simulink model "my_ODE_block"  (R2021b)
settings: Solver=VariableStepAuto  StartTime=0.0  StopTime=10.0  RelTol=1e-3
settings Model: Creator=Lorenzo  LastModifiedBy=Lorenzo

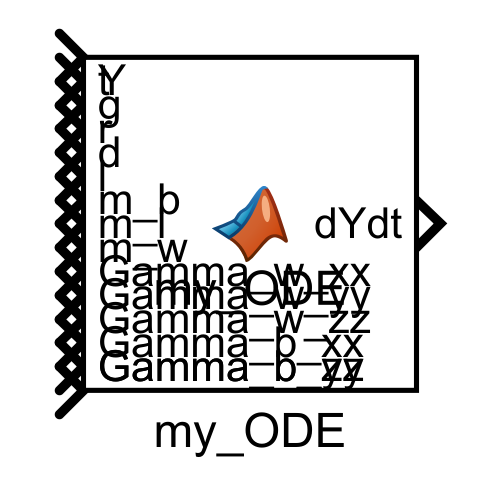
[thumbnail: Simulink's stored preview of the top-level diagram]
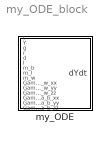
== system my_ODE_block ==
  my_ODE : MATLAB Function  TreatAsAtomicUnit=on

== matlab function my_ODE_block/my_ODE ==
  data: t input; dYdt output; Y input; g input; r input; d input; l input; m_b input; m_l input; m_w input; Gamma_w_xx input; Gamma_w_yy input; Gamma_w_zz input; Gamma_b_xx input; Gamma_b_yy input; Gamma_b_zz input
function dYdt = my_ODE(t,Y,g,r,d,l,m_b,m_l,m_w,Gamma_w_xx,Gamma_w_yy,Gamma_w_zz,Gamma_b_xx,Gamma_b_yy,Gamma_b_zz)
%#codegen

%    This function was generated by the Symbolic Math Toolbox version 9.0.
%    15-Jul-2022 11:26:44

t2 = Gamma_w_yy.^2;
t3 = Y(1);
t4 = Y(2);
t5 = Y(4);
t6 = Y(6);
t7 = d.^2;
t8 = d.^3;
t10 = l.^2;
t11 = m_w.^2;
t12 = m_w.^3;
t13 = r.^2;
t9 = t7.^2;
t14 = t13.^2;
t15 = abs(t4);
t16 = dirac(t4);
t17 = dirac(t5);
t18 = sign(t4);
t19 = sign(t5);
t20 = sin(t3);
t21 = t5.^2;
t22 = t6.^2;
t23 = l.*t4;
t26 = (d.*t5)./2.0;
t24 = t18.^2;
t25 = t19.^3;
t27 = -t26;
t28 = t6+t23;
t33 = t6+t26;
t29 = dirac(t28);
t30 = sign(t28);
t31 = abs(t28);
t34 = sign(t33);
t35 = t6+t27;
t36 = dirac(t33);
t32 = t30.^3;
t37 = sign(t35);
t38 = dirac(t35);
t39 = t6.*t29.*2.0;
t40 = t34.^3;
t42 = t23.*t29.*2.0;
t41 = t37.^3;
t43 = t32+t39+t42;
t44 = Gamma_b_zz.*Gamma_w_yy.*m_w.*t10.*t13.*t25.*t32.*t37.*t40.*4.0;
t46 = Gamma_w_yy.*Gamma_w_zz.*m_w.*t10.*t13.*t25.*t32.*t37.*t40.*8.0;
t49 = Gamma_b_zz.*t10.*t11.*t14.*t25.*t32.*t37.*t40.*4.0;
t51 = Gamma_b_yy.*Gamma_b_zz.*Gamma_w_yy.*t13.*t24.*t25.*t30.*t37.*t40.*4.0;
t53 = Gamma_b_yy.*Gamma_b_zz.*m_w.*t14.*t24.*t25.*t32.*t34.*t37.*4.0;
t54 = Gamma_b_yy.*Gamma_b_zz.*m_w.*t14.*t24.*t25.*t30.*t37.*t40.*4.0;
t56 = Gamma_b_zz.*Gamma_w_yy.*d.*m_w.*t5.*t10.*t13.*t25.*t32.*t36.*t37.*4.0;
t57 = Gamma_b_zz.*Gamma_w_yy.*d.*m_w.*t5.*t10.*t13.*t25.*t32.*t34.*t38.*4.0;
t58 = Gamma_w_zz.*t10.*t11.*t14.*t25.*t32.*t37.*t40.*8.0;
t60 = Gamma_b_yy.*Gamma_w_yy.*Gamma_w_zz.*t13.*t24.*t25.*t30.*t37.*t40.*8.0;
t63 = m_w.*t2.*t9.*t10.*t19.*t21.*t32.*t36.*t38.*4.0;
t64 = Gamma_b_zz.*Gamma_w_yy.*m_w.*t5.*t10.*t13.*t17.*t32.*t37.*t40.*8.0;
t66 = Gamma_b_zz.*Gamma_w_yy.*m_w.*t6.*t10.*t13.*t25.*t32.*t36.*t37.*8.0;
t67 = Gamma_b_zz.*Gamma_w_yy.*m_w.*t6.*t10.*t13.*t25.*t32.*t34.*t38.*8.0;
t68 = Gamma_w_yy.*Gamma_w_zz.*m_w.*t5.*t10.*t13.*t17.*t32.*t37.*t40.*1.6e+1;
t70 = Gamma_w_yy.*Gamma_w_zz.*m_w.*t6.*t10.*t13.*t25.*t32.*t36.*t37.*1.6e+1;
t71 = Gamma_w_yy.*Gamma_w_zz.*m_w.*t6.*t10.*t13.*t25.*t32.*t34.*t38.*1.6e+1;
t73 = m_w.*t2.*t5.*t8.*t10.*t19.*t32.*t38.*t40.*4.0;
t74 = Gamma_b_yy.*Gamma_w_zz.*m_w.*t14.*t24.*t25.*t32.*t34.*t37.*8.0;
t75 = Gamma_b_yy.*Gamma_w_zz.*m_w.*t14.*t24.*t25.*t30.*t37.*t40.*8.0;
t77 = Gamma_b_yy.*Gamma_b_zz.*m_w.*t5.*t14.*t17.*t24.*t32.*t34.*t37.*8.0;
t78 = Gamma_b_yy.*Gamma_b_zz.*m_w.*t5.*t14.*t17.*t24.*t30.*t37.*t40.*8.0;
t80 = Gamma_b_yy.*Gamma_b_zz.*m_w.*t6.*t14.*t24.*t25.*t29.*t34.*t37.*8.0;
t81 = Gamma_b_yy.*Gamma_b_zz.*m_w.*t6.*t14.*t24.*t25.*t30.*t36.*t37.*8.0;
t82 = Gamma_b_yy.*Gamma_b_zz.*m_w.*t6.*t14.*t24.*t25.*t30.*t34.*t38.*8.0;
t83 = Gamma_b_yy.*Gamma_w_zz.*m_w.*t5.*t14.*t17.*t24.*t32.*t34.*t37.*1.6e+1;
t84 = Gamma_b_yy.*Gamma_w_zz.*m_w.*t5.*t14.*t17.*t24.*t30.*t37.*t40.*1.6e+1;
t86 = Gamma_b_yy.*Gamma_w_zz.*m_w.*t6.*t14.*t24.*t25.*t29.*t34.*t37.*1.6e+1;
t87 = Gamma_b_yy.*Gamma_w_zz.*m_w.*t6.*t14.*t24.*t25.*t30.*t36.*t37.*1.6e+1;
t88 = Gamma_b_yy.*Gamma_w_zz.*m_w.*t6.*t14.*t24.*t25.*t30.*t34.*t38.*1.6e+1;
t90 = Gamma_w_yy.*Gamma_w_zz.*d.*m_w.*t5.*t10.*t13.*t25.*t32.*t36.*t37.*8.0;
t91 = Gamma_w_yy.*Gamma_w_zz.*d.*m_w.*t5.*t10.*t13.*t25.*t32.*t34.*t38.*8.0;
t92 = Gamma_b_zz.*d.*t5.*t10.*t11.*t14.*t25.*t32.*t36.*t37.*4.0;
t93 = Gamma_b_zz.*d.*t5.*t10.*t11.*t14.*t25.*t32.*t34.*t38.*4.0;
t94 = Gamma_b_yy.*Gamma_b_zz.*Gamma_w_yy.*d.*t5.*t13.*t24.*t25.*t30.*t36.*t37.*4.0;
t95 = Gamma_b_yy.*Gamma_b_zz.*Gamma_w_yy.*d.*t5.*t13.*t24.*t25.*t30.*t34.*t38.*4.0;
t96 = Gamma_b_yy.*Gamma_b_zz.*d.*m_w.*t5.*t14.*t24.*t25.*t30.*t36.*t37.*4.0;
t97 = Gamma_b_yy.*Gamma_b_zz.*d.*m_w.*t5.*t14.*t24.*t25.*t30.*t34.*t38.*4.0;
t98 = Gamma_b_yy.*Gamma_w_yy.*m_w.*t7.*t13.*t19.*t24.*t32.*t37.*t40;
t101 = m_w.*t2.*t7.*t10.*t19.*t22.*t32.*t36.*t38.*1.6e+1;
t104 = m_w.*t2.*t6.*t7.*t10.*t19.*t32.*t38.*t40.*8.0;
t105 = Gamma_b_zz.*t5.*t10.*t11.*t14.*t17.*t32.*t37.*t40.*8.0;
t107 = Gamma_b_zz.*t6.*t10.*t11.*t14.*t25.*t32.*t36.*t37.*8.0;
t108 = Gamma_b_zz.*t6.*t10.*t11.*t14.*t25.*t32.*t34.*t38.*8.0;
t109 = Gamma_w_zz.*t5.*t10.*t11.*t14.*t17.*t32.*t37.*t40.*1.6e+1;
t111 = Gamma_w_zz.*t6.*t10.*t11.*t14.*t25.*t32.*t36.*t37.*1.6e+1;
t112 = Gamma_w_zz.*t6.*t10.*t11.*t14.*t25.*t32.*t34.*t38.*1.6e+1;
t113 = Gamma_b_yy.*t2.*t9.*t19.*t21.*t24.*t30.*t36.*t38.*4.0;
t114 = Gamma_b_yy.*Gamma_b_zz.*Gamma_w_yy.*t5.*t13.*t17.*t24.*t30.*t37.*t40.*8.0;
t116 = Gamma_b_yy.*Gamma_b_zz.*Gamma_w_yy.*t6.*t13.*t24.*t25.*t30.*t36.*t37.*8.0;
t117 = Gamma_b_yy.*Gamma_b_zz.*Gamma_w_yy.*t6.*t13.*t24.*t25.*t30.*t34.*t38.*8.0;
t118 = Gamma_b_yy.*Gamma_w_yy.*Gamma_w_zz.*t5.*t13.*t17.*t24.*t30.*t37.*t40.*1.6e+1;
t120 = Gamma_b_yy.*Gamma_w_yy.*Gamma_w_zz.*t6.*t13.*t24.*t25.*t30.*t36.*t37.*1.6e+1;
t121 = Gamma_b_yy.*Gamma_w_yy.*Gamma_w_zz.*t6.*t13.*t24.*t25.*t30.*t34.*t38.*1.6e+1;
t123 = Gamma_b_yy.*t2.*t5.*t8.*t19.*t24.*t30.*t38.*t40.*4.0;
t124 = Gamma_b_zz.*Gamma_w_yy.*m_w.*t5.*t6.*t10.*t13.*t17.*t32.*t36.*t37.*1.6e+1;
t125 = Gamma_b_zz.*Gamma_w_yy.*m_w.*t5.*t6.*t10.*t13.*t17.*t32.*t34.*t38.*1.6e+1;
t126 = Gamma_w_yy.*Gamma_w_zz.*m_w.*t5.*t6.*t10.*t13.*t17.*t32.*t36.*t37.*3.2e+1;
t127 = Gamma_w_yy.*Gamma_w_zz.*m_w.*t5.*t6.*t10.*t13.*t17.*t32.*t34.*t38.*3.2e+1;
t129 = Gamma_b_zz.*Gamma_w_yy.*d.*m_w.*t10.*t13.*t17.*t21.*t32.*t36.*t37.*8.0;
t130 = Gamma_b_zz.*Gamma_w_yy.*d.*m_w.*t10.*t13.*t17.*t21.*t32.*t34.*t38.*8.0;
t131 = Gamma_w_yy.*Gamma_w_zz.*d.*m_w.*t10.*t13.*t17.*t21.*t32.*t36.*t37.*1.6e+1;
t132 = Gamma_w_yy.*Gamma_w_zz.*d.*m_w.*t10.*t13.*t17.*t21.*t32.*t34.*t38.*1.6e+1;
t133 = Gamma_b_zz.*t5.*t6.*t10.*t11.*t14.*t17.*t32.*t36.*t37.*1.6e+1;
t134 = Gamma_b_zz.*t5.*t6.*t10.*t11.*t14.*t17.*t32.*t34.*t38.*1.6e+1;
t135 = Gamma_w_zz.*t5.*t6.*t10.*t11.*t14.*t17.*t32.*t36.*t37.*3.2e+1;
t136 = Gamma_w_zz.*t5.*t6.*t10.*t11.*t14.*t17.*t32.*t34.*t38.*3.2e+1;
t138 = Gamma_b_zz.*d.*t10.*t11.*t14.*t17.*t21.*t32.*t36.*t37.*8.0;
t139 = Gamma_b_zz.*d.*t10.*t11.*t14.*t17.*t21.*t32.*t34.*t38.*8.0;
t140 = Gamma_w_zz.*d.*t10.*t11.*t14.*t17.*t21.*t32.*t36.*t37.*1.6e+1;
t141 = Gamma_w_zz.*d.*t10.*t11.*t14.*t17.*t21.*t32.*t34.*t38.*1.6e+1;
t143 = Gamma_w_zz.*d.*t5.*t10.*t11.*t14.*t25.*t32.*t36.*t37.*8.0;
t144 = Gamma_w_zz.*d.*t5.*t10.*t11.*t14.*t25.*t32.*t34.*t38.*8.0;
t145 = Gamma_b_yy.*Gamma_b_zz.*Gamma_w_yy.*t5.*t6.*t13.*t17.*t24.*t30.*t36.*t37.*1.6e+1;
t146 = Gamma_b_yy.*Gamma_b_zz.*Gamma_w_yy.*t5.*t6.*t13.*t17.*t24.*t30.*t34.*t38.*1.6e+1;
t147 = Gamma_b_yy.*Gamma_w_yy.*Gamma_w_zz.*t5.*t6.*t13.*t17.*t24.*t30.*t36.*t37.*3.2e+1;
t148 = Gamma_b_yy.*Gamma_w_yy.*Gamma_w_zz.*t5.*t6.*t13.*t17.*t24.*t30.*t34.*t38.*3.2e+1;
t149 = t9.*t10.*t12.*t14.*t19.*t21.*t32.*t36.*t38.*4.0;
t150 = Gamma_b_yy.*Gamma_b_zz.*Gamma_w_yy.*d.*t13.*t17.*t21.*t24.*t30.*t36.*t37.*8.0;
t151 = Gamma_b_yy.*Gamma_b_zz.*Gamma_w_yy.*d.*t13.*t17.*t21.*t24.*t30.*t34.*t38.*8.0;
t152 = Gamma_b_yy.*Gamma_w_yy.*Gamma_w_zz.*d.*t13.*t17.*t21.*t24.*t30.*t36.*t37.*1.6e+1;
t153 = Gamma_b_yy.*Gamma_w_yy.*Gamma_w_zz.*d.*t13.*t17.*t21.*t24.*t30.*t34.*t38.*1.6e+1;
t155 = t5.*t8.*t10.*t12.*t14.*t19.*t32.*t38.*t40.*4.0;
t156 = Gamma_b_yy.*Gamma_b_zz.*Gamma_w_yy.*t13.*t15.*t16.*t25.*t30.*t37.*t40.*8.0;
t158 = Gamma_b_yy.*Gamma_w_yy.*Gamma_w_zz.*t13.*t15.*t16.*t25.*t30.*t37.*t40.*1.6e+1;
t161 = Gamma_b_yy.*Gamma_w_yy.*Gamma_w_zz.*d.*t5.*t13.*t24.*t25.*t30.*t36.*t37.*8.0;
t162 = Gamma_b_yy.*Gamma_w_yy.*Gamma_w_zz.*d.*t5.*t13.*t24.*t25.*t30.*t34.*t38.*8.0;
t163 = Gamma_b_yy.*Gamma_b_zz.*m_w.*t5.*t6.*t14.*t17.*t24.*t29.*t34.*t37.*1.6e+1;
t164 = Gamma_b_yy.*Gamma_b_zz.*m_w.*t5.*t6.*t14.*t17.*t24.*t30.*t36.*t37.*1.6e+1;
t165 = Gamma_b_yy.*Gamma_b_zz.*m_w.*t5.*t6.*t14.*t17.*t24.*t30.*t34.*t38.*1.6e+1;
t166 = Gamma_b_yy.*Gamma_w_zz.*m_w.*t5.*t6.*t14.*t17.*t24.*t29.*t34.*t37.*3.2e+1;
t167 = Gamma_b_yy.*Gamma_w_zz.*m_w.*t5.*t6.*t14.*t17.*t24.*t30.*t36.*t37.*3.2e+1;
t168 = Gamma_b_yy.*Gamma_w_zz.*m_w.*t5.*t6.*t14.*t17.*t24.*t30.*t34.*t38.*3.2e+1;
t169 = Gamma_b_yy.*Gamma_b_zz.*d.*m_w.*t14.*t17.*t21.*t24.*t30.*t36.*t37.*8.0;
t170 = Gamma_b_yy.*Gamma_b_zz.*d.*m_w.*t14.*t17.*t21.*t24.*t30.*t34.*t38.*8.0;
t171 = Gamma_b_yy.*Gamma_w_zz.*d.*m_w.*t14.*t17.*t21.*t24.*t30.*t36.*t37.*1.6e+1;
t172 = Gamma_b_yy.*Gamma_w_zz.*d.*m_w.*t14.*t17.*t21.*t24.*t30.*t34.*t38.*1.6e+1;
t173 = Gamma_b_yy.*Gamma_b_zz.*m_w.*t14.*t15.*t16.*t25.*t32.*t34.*t37.*8.0;
t174 = Gamma_b_yy.*Gamma_b_zz.*m_w.*t14.*t15.*t16.*t25.*t30.*t37.*t40.*8.0;
t176 = Gamma_b_yy.*Gamma_w_zz.*m_w.*t14.*t15.*t16.*t25.*t32.*t34.*t37.*1.6e+1;
t177 = Gamma_b_yy.*Gamma_w_zz.*m_w.*t14.*t15.*t16.*t25.*t30.*t37.*t40.*1.6e+1;
t180 = Gamma_b_yy.*Gamma_w_zz.*d.*m_w.*t5.*t14.*t24.*t25.*t30.*t36.*t37.*8.0;
t181 = Gamma_b_yy.*Gamma_w_zz.*d.*m_w.*t5.*t14.*t24.*t25.*t30.*t34.*t38.*8.0;
t182 = Gamma_b_yy.*Gamma_b_zz.*m_w.*t14.*t23.*t24.*t25.*t29.*t34.*t37.*8.0;
t183 = Gamma_b_yy.*Gamma_w_zz.*m_w.*t14.*t23.*t24.*t25.*t29.*t34.*t37.*1.6e+1;
t184 = Gamma_b_yy.*t7.*t11.*t14.*t19.*t24.*t32.*t37.*t40;
t186 = Gamma_b_yy.*Gamma_w_yy.*m_w.*t5.*t8.*t13.*t19.*t24.*t32.*t36.*t37;
t187 = Gamma_b_yy.*Gamma_w_yy.*m_w.*t5.*t8.*t13.*t19.*t24.*t32.*t34.*t38;
t189 = Gamma_b_yy.*t2.*t7.*t19.*t22.*t24.*t30.*t36.*t38.*1.6e+1;
t192 = Gamma_b_yy.*t2.*t6.*t7.*t19.*t24.*t30.*t38.*t40.*8.0;
t199 = t7.*t10.*t12.*t14.*t19.*t22.*t32.*t36.*t38.*1.6e+1;
t205 = t6.*t7.*t10.*t12.*t14.*t19.*t32.*t38.*t40.*8.0;
t212 = Gamma_b_yy.*Gamma_b_zz.*Gamma_w_yy.*t5.*t13.*t15.*t16.*t17.*t30.*t37.*t40.*1.6e+1;
t214 = Gamma_b_yy.*Gamma_b_zz.*Gamma_w_yy.*t6.*t13.*t15.*t16.*t25.*t30.*t36.*t37.*1.6e+1;
t215 = Gamma_b_yy.*Gamma_b_zz.*Gamma_w_yy.*t6.*t13.*t15.*t16.*t25.*t30.*t34.*t38.*1.6e+1;
t216 = Gamma_b_yy.*Gamma_w_yy.*Gamma_w_zz.*t5.*t13.*t15.*t16.*t17.*t30.*t37.*t40.*3.2e+1;
t218 = Gamma_b_yy.*Gamma_w_yy.*Gamma_w_zz.*t6.*t13.*t15.*t16.*t25.*t30.*t36.*t37.*3.2e+1;
t219 = Gamma_b_yy.*Gamma_w_yy.*Gamma_w_zz.*t6.*t13.*t15.*t16.*t25.*t30.*t34.*t38.*3.2e+1;
t221 = Gamma_b_yy.*Gamma_b_zz.*m_w.*t5.*t14.*t15.*t16.*t17.*t32.*t34.*t37.*1.6e+1;
t222 = Gamma_b_yy.*Gamma_b_zz.*m_w.*t5.*t14.*t15.*t16.*t17.*t30.*t37.*t40.*1.6e+1;
t224 = Gamma_b_yy.*Gamma_b_zz.*m_w.*t6.*t14.*t15.*t16.*t25.*t29.*t34.*t37.*1.6e+1;
t225 = Gamma_b_yy.*Gamma_b_zz.*m_w.*t6.*t14.*t15.*t16.*t25.*t30.*t36.*t37.*1.6e+1;
t226 = Gamma_b_yy.*Gamma_b_zz.*m_w.*t6.*t14.*t15.*t16.*t25.*t30.*t34.*t38.*1.6e+1;
t227 = Gamma_b_yy.*Gamma_w_zz.*m_w.*t5.*t14.*t15.*t16.*t17.*t32.*t34.*t37.*3.2e+1;
t228 = Gamma_b_yy.*Gamma_w_zz.*m_w.*t5.*t14.*t15.*t16.*t17.*t30.*t37.*t40.*3.2e+1;
t230 = Gamma_b_yy.*Gamma_w_zz.*m_w.*t6.*t14.*t15.*t16.*t25.*t29.*t34.*t37.*3.2e+1;
t231 = Gamma_b_yy.*Gamma_w_zz.*m_w.*t6.*t14.*t15.*t16.*t25.*t30.*t36.*t37.*3.2e+1;
t232 = Gamma_b_yy.*Gamma_w_zz.*m_w.*t6.*t14.*t15.*t16.*t25.*t30.*t34.*t38.*3.2e+1;
t233 = Gamma_b_yy.*Gamma_w_yy.*m_w.*t7.*t13.*t19.*t22.*t24.*t29.*t36.*t37.*4.0;
t234 = Gamma_b_yy.*Gamma_w_yy.*m_w.*t7.*t13.*t19.*t22.*t24.*t29.*t34.*t38.*4.0;
t235 = Gamma_b_yy.*Gamma_b_zz.*m_w.*t5.*t14.*t17.*t23.*t24.*t29.*t34.*t37.*1.6e+1;
t236 = Gamma_b_yy.*Gamma_w_zz.*m_w.*t5.*t14.*t17.*t23.*t24.*t29.*t34.*t37.*3.2e+1;
t237 = Gamma_b_yy.*Gamma_w_yy.*m_w.*t7.*t13.*t19.*t24.*t37.*t39.*t40;
t239 = Gamma_b_yy.*Gamma_w_yy.*m_w.*t6.*t7.*t13.*t19.*t24.*t32.*t36.*t37.*2.0;
t240 = Gamma_b_yy.*Gamma_w_yy.*m_w.*t6.*t7.*t13.*t19.*t24.*t32.*t34.*t38.*2.0;
t241 = Gamma_b_yy.*t5.*t8.*t11.*t14.*t19.*t24.*t32.*t36.*t37;
t242 = Gamma_b_yy.*t5.*t8.*t11.*t14.*t19.*t24.*t32.*t34.*t38;
t243 = Gamma_b_yy.*Gamma_b_zz.*d.*m_w.*t14.*t15.*t16.*t17.*t21.*t30.*t36.*t37.*1.6e+1;
t244 = Gamma_b_yy.*Gamma_b_zz.*d.*m_w.*t14.*t15.*t16.*t17.*t21.*t30.*t34.*t38.*1.6e+1;
t245 = Gamma_b_yy.*Gamma_w_zz.*d.*m_w.*t14.*t15.*t16.*t17.*t21.*t30.*t36.*t37.*3.2e+1;
t246 = Gamma_b_yy.*Gamma_w_zz.*d.*m_w.*t14.*t15.*t16.*t17.*t21.*t30.*t34.*t38.*3.2e+1;
t247 = Gamma_b_yy.*Gamma_w_yy.*m_w.*t5.*t8.*t13.*t19.*t24.*t36.*t37.*t39;
t248 = Gamma_b_yy.*Gamma_w_yy.*m_w.*t5.*t8.*t13.*t19.*t24.*t34.*t38.*t39;
t249 = Gamma_b_yy.*Gamma_b_zz.*d.*m_w.*t5.*t14.*t15.*t16.*t25.*t30.*t36.*t37.*8.0;
t250 = Gamma_b_yy.*Gamma_b_zz.*d.*m_w.*t5.*t14.*t15.*t16.*t25.*t30.*t34.*t38.*8.0;
t251 = Gamma_b_yy.*Gamma_w_zz.*d.*m_w.*t5.*t14.*t15.*t16.*t25.*t30.*t36.*t37.*1.6e+1;
t252 = Gamma_b_yy.*Gamma_w_zz.*d.*m_w.*t5.*t14.*t15.*t16.*t25.*t30.*t34.*t38.*1.6e+1;
t253 = Gamma_b_yy.*Gamma_b_zz.*m_w.*t14.*t15.*t16.*t23.*t25.*t29.*t34.*t37.*1.6e+1;
t254 = Gamma_b_yy.*Gamma_w_zz.*m_w.*t14.*t15.*t16.*t23.*t25.*t29.*t34.*t37.*3.2e+1;
t255 = Gamma_b_yy.*Gamma_w_yy.*m_w.*t7.*t13.*t15.*t16.*t19.*t32.*t37.*t40.*2.0;
t257 = Gamma_b_yy.*Gamma_w_yy.*m_w.*t7.*t13.*t19.*t24.*t37.*t40.*t42;
t259 = Gamma_w_yy.*t9.*t10.*t11.*t13.*t19.*t21.*t32.*t36.*t38.*8.0;
t260 = Gamma_w_yy.*t7.*t10.*t11.*t13.*t19.*t22.*t32.*t36.*t38.*3.2e+1;
t262 = Gamma_w_yy.*t5.*t8.*t10.*t11.*t13.*t19.*t32.*t38.*t40.*8.0;
t264 = Gamma_w_yy.*t6.*t7.*t10.*t11.*t13.*t19.*t32.*t38.*t40.*1.6e+1;
t265 = Gamma_b_yy.*t2.*t9.*t15.*t16.*t19.*t21.*t30.*t36.*t38.*8.0;
t266 = Gamma_b_yy.*t2.*t7.*t15.*t16.*t19.*t22.*t30.*t36.*t38.*3.2e+1;
t268 = Gamma_b_yy.*t2.*t5.*t8.*t15.*t16.*t19.*t30.*t38.*t40.*8.0;
t270 = Gamma_b_yy.*t2.*t6.*t7.*t15.*t16.*t19.*t30.*t38.*t40.*1.6e+1;
t271 = Gamma_b_yy.*Gamma_w_yy.*m_w.*t9.*t13.*t19.*t21.*t24.*t30.*t36.*t38.*8.0;
t272 = Gamma_b_yy.*Gamma_w_yy.*m_w.*t7.*t13.*t19.*t22.*t24.*t30.*t36.*t38.*3.2e+1;
t275 = Gamma_b_yy.*Gamma_w_yy.*m_w.*t5.*t8.*t13.*t19.*t24.*t30.*t38.*t40.*8.0;
t277 = Gamma_b_yy.*Gamma_w_yy.*m_w.*t6.*t7.*t13.*t19.*t24.*t30.*t38.*t40.*1.6e+1;
t278 = Gamma_b_yy.*t7.*t11.*t14.*t19.*t22.*t24.*t29.*t36.*t37.*4.0;
t279 = Gamma_b_yy.*t7.*t11.*t14.*t19.*t22.*t24.*t29.*t34.*t38.*4.0;
t280 = Gamma_b_yy.*t9.*t11.*t14.*t19.*t21.*t24.*t30.*t36.*t38.*4.0;
t281 = Gamma_b_yy.*Gamma_b_zz.*Gamma_w_yy.*t5.*t6.*t13.*t15.*t16.*t17.*t30.*t36.*t37.*3.2e+1;
t282 = Gamma_b_yy.*Gamma_b_zz.*Gamma_w_yy.*t5.*t6.*t13.*t15.*t16.*t17.*t30.*t34.*t38.*3.2e+1;
t283 = Gamma_b_yy.*Gamma_b_zz.*Gamma_w_yy.*d.*t13.*t15.*t16.*t17.*t21.*t30.*t36.*t37.*1.6e+1;
t284 = Gamma_b_yy.*Gamma_b_zz.*Gamma_w_yy.*d.*t13.*t15.*t16.*t17.*t21.*t30.*t34.*t38.*1.6e+1;
t285 = Gamma_b_yy.*Gamma_w_yy.*Gamma_w_zz.*d.*t13.*t15.*t16.*t17.*t21.*t30.*t36.*t37.*3.2e+1;
t286 = Gamma_b_yy.*Gamma_w_yy.*Gamma_w_zz.*d.*t13.*t15.*t16.*t17.*t21.*t30.*t34.*t38.*3.2e+1;
t287 = Gamma_b_yy.*t7.*t11.*t14.*t19.*t24.*t37.*t39.*t40;
t289 = Gamma_b_yy.*t6.*t7.*t11.*t14.*t19.*t24.*t32.*t36.*t37.*2.0;
t290 = Gamma_b_yy.*t6.*t7.*t11.*t14.*t19.*t24.*t32.*t34.*t38.*2.0;
t292 = Gamma_b_yy.*t5.*t8.*t11.*t14.*t19.*t24.*t30.*t38.*t40.*4.0;
t293 = Gamma_b_yy.*Gamma_b_zz.*Gamma_w_yy.*d.*t5.*t13.*t15.*t16.*t25.*t30.*t36.*t37.*8.0;
t294 = Gamma_b_yy.*Gamma_b_zz.*Gamma_w_yy.*d.*t5.*t13.*t15.*t16.*t25.*t30.*t34.*t38.*8.0;
t295 = Gamma_b_yy.*Gamma_w_yy.*Gamma_w_zz.*d.*t5.*t13.*t15.*t16.*t25.*t30.*t36.*t37.*1.6e+1;
t296 = Gamma_b_yy.*Gamma_w_yy.*Gamma_w_zz.*d.*t5.*t13.*t15.*t16.*t25.*t30.*t34.*t38.*1.6e+1;
t297 = Gamma_b_yy.*Gamma_b_zz.*m_w.*t5.*t6.*t14.*t15.*t16.*t17.*t29.*t34.*t37.*3.2e+1;
t298 = Gamma_b_yy.*Gamma_b_zz.*m_w.*t5.*t6.*t14.*t15.*t16.*t17.*t30.*t36.*t37.*3.2e+1;
t299 = Gamma_b_yy.*Gamma_b_zz.*m_w.*t5.*t6.*t14.*t15.*t16.*t17.*t30.*t34.*t38.*3.2e+1;
t302 = Gamma_b_yy.*Gamma_w_yy.*m_w.*t5.*t6.*t8.*t13.*t19.*t24.*t29.*t34.*t38.*-2.0;
t306 = Gamma_b_yy.*t5.*t8.*t11.*t14.*t19.*t24.*t36.*t37.*t39;
t307 = Gamma_b_yy.*t5.*t8.*t11.*t14.*t19.*t24.*t34.*t38.*t39;
t308 = Gamma_b_yy.*t7.*t11.*t14.*t15.*t16.*t19.*t32.*t37.*t40.*2.0;
t310 = Gamma_b_yy.*t7.*t11.*t14.*t19.*t24.*t37.*t40.*t42;
t312 = Gamma_b_yy.*Gamma_b_zz.*m_w.*t5.*t14.*t15.*t16.*t17.*t23.*t29.*t34.*t37.*3.2e+1;
t314 = Gamma_b_yy.*Gamma_w_yy.*m_w.*t5.*t8.*t13.*t15.*t16.*t19.*t32.*t36.*t37.*2.0;
t315 = Gamma_b_yy.*Gamma_w_yy.*m_w.*t5.*t8.*t13.*t15.*t16.*t19.*t32.*t34.*t38.*2.0;
t316 = Gamma_b_yy.*Gamma_w_yy.*m_w.*t6.*t7.*t13.*t15.*t16.*t19.*t29.*t37.*t40.*4.0;
t318 = Gamma_b_yy.*Gamma_w_yy.*m_w.*t6.*t7.*t13.*t15.*t16.*t19.*t32.*t36.*t37.*4.0;
t319 = Gamma_b_yy.*Gamma_w_yy.*m_w.*t6.*t7.*t13.*t15.*t16.*t19.*t32.*t34.*t38.*4.0;
t320 = Gamma_b_yy.*Gamma_w_yy.*m_w.*t5.*t8.*t13.*t19.*t24.*t36.*t37.*t42;
t321 = Gamma_b_yy.*Gamma_w_yy.*m_w.*t5.*t8.*t13.*t19.*t24.*t34.*t38.*t42;
t322 = Gamma_b_yy.*Gamma_w_yy.*m_w.*t6.*t7.*t13.*t19.*t23.*t24.*t29.*t36.*t37.*4.0;
t323 = Gamma_b_yy.*Gamma_w_yy.*m_w.*t6.*t7.*t13.*t19.*t23.*t24.*t29.*t34.*t38.*4.0;
t330 = Gamma_b_yy.*t7.*t11.*t14.*t19.*t22.*t24.*t30.*t36.*t38.*1.6e+1;
t331 = Gamma_b_yy.*Gamma_w_yy.*Gamma_w_zz.*t5.*t6.*t13.*t15.*t16.*t17.*t30.*t36.*t37.*6.4e+1;
t332 = Gamma_b_yy.*Gamma_w_yy.*Gamma_w_zz.*t5.*t6.*t13.*t15.*t16.*t17.*t30.*t34.*t38.*6.4e+1;
t338 = Gamma_b_yy.*t6.*t7.*t11.*t14.*t19.*t24.*t30.*t38.*t40.*8.0;
t341 = Gamma_b_yy.*Gamma_w_zz.*m_w.*t5.*t6.*t14.*t15.*t16.*t17.*t29.*t34.*t37.*6.4e+1;
t342 = Gamma_b_yy.*Gamma_w_zz.*m_w.*t5.*t6.*t14.*t15.*t16.*t17.*t30.*t36.*t37.*6.4e+1;
t343 = Gamma_b_yy.*Gamma_w_zz.*m_w.*t5.*t6.*t14.*t15.*t16.*t17.*t30.*t34.*t38.*6.4e+1;
t344 = Gamma_b_yy.*t5.*t6.*t8.*t11.*t14.*t19.*t24.*t29.*t34.*t38.*-2.0;
t346 = Gamma_b_yy.*Gamma_w_yy.*m_w.*t7.*t13.*t15.*t16.*t19.*t22.*t29.*t36.*t37.*8.0;
t347 = Gamma_b_yy.*Gamma_w_yy.*m_w.*t7.*t13.*t15.*t16.*t19.*t22.*t29.*t34.*t38.*8.0;
t348 = Gamma_b_yy.*Gamma_w_yy.*m_w.*t9.*t13.*t15.*t16.*t19.*t21.*t30.*t36.*t38.*1.6e+1;
t349 = Gamma_b_yy.*Gamma_w_zz.*m_w.*t5.*t14.*t15.*t16.*t17.*t23.*t29.*t34.*t37.*6.4e+1;
t352 = Gamma_b_yy.*Gamma_w_yy.*m_w.*t5.*t8.*t13.*t15.*t16.*t19.*t30.*t38.*t40.*1.6e+1;
t354 = Gamma_b_yy.*Gamma_w_yy.*m_w.*t6.*t7.*t13.*t15.*t16.*t19.*t30.*t38.*t40.*3.2e+1;
t355 = Gamma_b_yy.*Gamma_w_yy.*m_w.*t5.*t8.*t13.*t19.*t23.*t24.*t29.*t34.*t38.*-2.0;
t356 = Gamma_b_yy.*t5.*t8.*t11.*t14.*t15.*t16.*t19.*t32.*t36.*t37.*2.0;
t357 = Gamma_b_yy.*t5.*t8.*t11.*t14.*t15.*t16.*t19.*t32.*t34.*t38.*2.0;
t358 = Gamma_b_yy.*t6.*t7.*t11.*t14.*t15.*t16.*t19.*t29.*t37.*t40.*4.0;
t360 = Gamma_b_yy.*t6.*t7.*t11.*t14.*t15.*t16.*t19.*t32.*t36.*t37.*4.0;
t361 = Gamma_b_yy.*t6.*t7.*t11.*t14.*t15.*t16.*t19.*t32.*t34.*t38.*4.0;
t362 = Gamma_b_yy.*t5.*t8.*t11.*t14.*t19.*t24.*t36.*t37.*t42;
t363 = Gamma_b_yy.*t5.*t8.*t11.*t14.*t19.*t24.*t34.*t38.*t42;
t364 = Gamma_b_yy.*t6.*t7.*t11.*t14.*t19.*t23.*t24.*t29.*t36.*t37.*4.0;
t365 = Gamma_b_yy.*t6.*t7.*t11.*t14.*t19.*t23.*t24.*t29.*t34.*t38.*4.0;
t366 = Gamma_b_yy.*Gamma_w_yy.*m_w.*t5.*t6.*t8.*t13.*t15.*t16.*t19.*t29.*t36.*t37.*4.0;
t367 = Gamma_b_yy.*Gamma_w_yy.*m_w.*t5.*t6.*t8.*t13.*t15.*t16.*t19.*t29.*t34.*t38.*4.0;
t368 = Gamma_b_yy.*Gamma_w_yy.*m_w.*t7.*t13.*t15.*t16.*t19.*t23.*t29.*t37.*t40.*4.0;
t370 = Gamma_b_yy.*Gamma_w_yy.*m_w.*t5.*t8.*t13.*t15.*t16.*t19.*t23.*t29.*t36.*t37.*4.0;
t371 = Gamma_b_yy.*Gamma_w_yy.*m_w.*t5.*t8.*t13.*t15.*t16.*t19.*t23.*t29.*t34.*t38.*4.0;
t373 = Gamma_b_yy.*Gamma_w_yy.*m_w.*t7.*t13.*t15.*t16.*t19.*t22.*t30.*t36.*t38.*6.4e+1;
t375 = Gamma_b_yy.*t7.*t11.*t14.*t15.*t16.*t19.*t22.*t29.*t36.*t37.*8.0;
t376 = Gamma_b_yy.*t7.*t11.*t14.*t15.*t16.*t19.*t22.*t29.*t34.*t38.*8.0;
t377 = Gamma_b_yy.*t9.*t11.*t14.*t15.*t16.*t19.*t21.*t30.*t36.*t38.*8.0;
t378 = Gamma_b_yy.*t7.*t11.*t14.*t15.*t16.*t19.*t22.*t30.*t36.*t38.*3.2e+1;
t381 = Gamma_b_yy.*t5.*t8.*t11.*t14.*t15.*t16.*t19.*t30.*t38.*t40.*8.0;
t383 = Gamma_b_yy.*t6.*t7.*t11.*t14.*t15.*t16.*t19.*t30.*t38.*t40.*1.6e+1;
t384 = Gamma_b_yy.*t5.*t8.*t11.*t14.*t19.*t23.*t24.*t29.*t34.*t38.*-2.0;
t386 = Gamma_b_yy.*t5.*t6.*t8.*t11.*t14.*t15.*t16.*t19.*t29.*t36.*t37.*4.0;
t387 = Gamma_b_yy.*t5.*t6.*t8.*t11.*t14.*t15.*t16.*t19.*t29.*t34.*t38.*4.0;
t388 = Gamma_b_yy.*t7.*t11.*t14.*t15.*t16.*t19.*t23.*t29.*t37.*t40.*4.0;
t391 = Gamma_b_yy.*Gamma_w_yy.*m_w.*t6.*t7.*t13.*t15.*t16.*t19.*t23.*t29.*t36.*t37.*8.0;
t392 = Gamma_b_yy.*Gamma_w_yy.*m_w.*t6.*t7.*t13.*t15.*t16.*t19.*t23.*t29.*t34.*t38.*8.0;
t393 = Gamma_b_yy.*t5.*t8.*t11.*t14.*t15.*t16.*t19.*t23.*t29.*t36.*t37.*4.0;
t394 = Gamma_b_yy.*t5.*t8.*t11.*t14.*t15.*t16.*t19.*t23.*t29.*t34.*t38.*4.0;
t399 = Gamma_b_yy.*t6.*t7.*t11.*t14.*t15.*t16.*t19.*t23.*t29.*t36.*t37.*8.0;
t400 = Gamma_b_yy.*t6.*t7.*t11.*t14.*t15.*t16.*t19.*t23.*t29.*t34.*t38.*8.0;
t401 = Gamma_b_zz.*Gamma_w_yy.*m_w.*t10.*t13.*t25.*t29.*t30.*t31.*t37.*t40.*8.0;
t403 = Gamma_w_yy.*Gamma_w_zz.*m_w.*t10.*t13.*t25.*t29.*t30.*t31.*t37.*t40.*1.6e+1;
t406 = Gamma_b_zz.*t10.*t11.*t14.*t25.*t29.*t30.*t31.*t37.*t40.*8.0;
t408 = Gamma_w_zz.*t10.*t11.*t14.*t25.*t29.*t30.*t31.*t37.*t40.*1.6e+1;
t410 = Gamma_b_zz.*Gamma_w_yy.*m_w.*t5.*t10.*t13.*t17.*t29.*t30.*t31.*t37.*t40.*1.6e+1;
t412 = Gamma_b_zz.*Gamma_w_yy.*m_w.*t6.*t10.*t13.*t25.*t29.*t30.*t31.*t36.*t37.*1.6e+1;
t413 = Gamma_b_zz.*Gamma_w_yy.*m_w.*t6.*t10.*t13.*t25.*t29.*t30.*t31.*t34.*t38.*1.6e+1;
t414 = Gamma_w_yy.*Gamma_w_zz.*m_w.*t5.*t10.*t13.*t17.*t29.*t30.*t31.*t37.*t40.*3.2e+1;
t416 = Gamma_w_yy.*Gamma_w_zz.*m_w.*t6.*t10.*t13.*t25.*t29.*t30.*t31.*t36.*t37.*3.2e+1;
t417 = Gamma_w_yy.*Gamma_w_zz.*m_w.*t6.*t10.*t13.*t25.*t29.*t30.*t31.*t34.*t38.*3.2e+1;
t418 = m_w.*t2.*t9.*t10.*t19.*t21.*t29.*t30.*t31.*t36.*t38.*8.0;
t419 = m_w.*t2.*t7.*t10.*t19.*t22.*t29.*t30.*t31.*t36.*t38.*3.2e+1;
t421 = m_w.*t2.*t5.*t8.*t10.*t19.*t29.*t30.*t31.*t38.*t40.*8.0;
t423 = m_w.*t2.*t6.*t7.*t10.*t19.*t29.*t30.*t31.*t38.*t40.*1.6e+1;
t424 = Gamma_b_zz.*t5.*t10.*t11.*t14.*t17.*t29.*t30.*t31.*t37.*t40.*1.6e+1;
t426 = Gamma_b_zz.*t6.*t10.*t11.*t14.*t25.*t29.*t30.*t31.*t36.*t37.*1.6e+1;
t427 = Gamma_b_zz.*t6.*t10.*t11.*t14.*t25.*t29.*t30.*t31.*t34.*t38.*1.6e+1;
t428 = Gamma_w_zz.*t5.*t10.*t11.*t14.*t17.*t29.*t30.*t31.*t37.*t40.*3.2e+1;
t430 = Gamma_w_zz.*t6.*t10.*t11.*t14.*t25.*t29.*t30.*t31.*t36.*t37.*3.2e+1;
t431 = Gamma_w_zz.*t6.*t10.*t11.*t14.*t25.*t29.*t30.*t31.*t34.*t38.*3.2e+1;
t432 = Gamma_b_zz.*Gamma_w_yy.*m_w.*t5.*t6.*t10.*t13.*t17.*t29.*t30.*t31.*t36.*t37.*3.2e+1;
t433 = Gamma_b_zz.*Gamma_w_yy.*m_w.*t5.*t6.*t10.*t13.*t17.*t29.*t30.*t31.*t34.*t38.*3.2e+1;
t434 = Gamma_b_zz.*Gamma_w_yy.*d.*m_w.*t10.*t13.*t17.*t21.*t29.*t30.*t31.*t36.*t37.*1.6e+1;
t435 = Gamma_b_zz.*Gamma_w_yy.*d.*m_w.*t10.*t13.*t17.*t21.*t29.*t30.*t31.*t34.*t38.*1.6e+1;
t436 = Gamma_w_yy.*Gamma_w_zz.*d.*m_w.*t10.*t13.*t17.*t21.*t29.*t30.*t31.*t36.*t37.*3.2e+1;
t437 = Gamma_w_yy.*Gamma_w_zz.*d.*m_w.*t10.*t13.*t17.*t21.*t29.*t30.*t31.*t34.*t38.*3.2e+1;
t438 = Gamma_b_zz.*Gamma_w_yy.*d.*m_w.*t5.*t10.*t13.*t25.*t29.*t30.*t31.*t36.*t37.*8.0;
t439 = Gamma_b_zz.*Gamma_w_yy.*d.*m_w.*t5.*t10.*t13.*t25.*t29.*t30.*t31.*t34.*t38.*8.0;
t440 = Gamma_w_yy.*Gamma_w_zz.*d.*m_w.*t5.*t10.*t13.*t25.*t29.*t30.*t31.*t36.*t37.*1.6e+1;
t441 = Gamma_w_yy.*Gamma_w_zz.*d.*m_w.*t5.*t10.*t13.*t25.*t29.*t30.*t31.*t34.*t38.*1.6e+1;
t444 = Gamma_w_yy.*Gamma_w_zz.*m_w.*t5.*t6.*t10.*t13.*t17.*t29.*t30.*t31.*t36.*t37.*6.4e+1;
t445 = Gamma_w_yy.*Gamma_w_zz.*m_w.*t5.*t6.*t10.*t13.*t17.*t29.*t30.*t31.*t34.*t38.*6.4e+1;
t449 = Gamma_b_zz.*t5.*t6.*t10.*t11.*t14.*t17.*t29.*t30.*t31.*t36.*t37.*3.2e+1;
t450 = Gamma_b_zz.*t5.*t6.*t10.*t11.*t14.*t17.*t29.*t30.*t31.*t34.*t38.*3.2e+1;
t453 = Gamma_b_zz.*d.*t10.*t11.*t14.*t17.*t21.*t29.*t30.*t31.*t36.*t37.*1.6e+1;
t454 = Gamma_b_zz.*d.*t10.*t11.*t14.*t17.*t21.*t29.*t30.*t31.*t34.*t38.*1.6e+1;
t455 = Gamma_w_zz.*d.*t10.*t11.*t14.*t17.*t21.*t29.*t30.*t31.*t36.*t37.*3.2e+1;
t456 = Gamma_w_zz.*d.*t10.*t11.*t14.*t17.*t21.*t29.*t30.*t31.*t34.*t38.*3.2e+1;
t457 = Gamma_b_zz.*d.*t5.*t10.*t11.*t14.*t25.*t29.*t30.*t31.*t36.*t37.*8.0;
t458 = Gamma_b_zz.*d.*t5.*t10.*t11.*t14.*t25.*t29.*t30.*t31.*t34.*t38.*8.0;
t459 = Gamma_w_zz.*d.*t5.*t10.*t11.*t14.*t25.*t29.*t30.*t31.*t36.*t37.*1.6e+1;
t460 = Gamma_w_zz.*d.*t5.*t10.*t11.*t14.*t25.*t29.*t30.*t31.*t34.*t38.*1.6e+1;
t461 = Gamma_w_zz.*t5.*t6.*t10.*t11.*t14.*t17.*t29.*t30.*t31.*t36.*t37.*6.4e+1;
t462 = Gamma_w_zz.*t5.*t6.*t10.*t11.*t14.*t17.*t29.*t30.*t31.*t34.*t38.*6.4e+1;
t467 = t9.*t10.*t12.*t14.*t19.*t21.*t29.*t30.*t31.*t36.*t38.*8.0;
t468 = t7.*t10.*t12.*t14.*t19.*t22.*t29.*t30.*t31.*t36.*t38.*3.2e+1;
t471 = t5.*t8.*t10.*t12.*t14.*t19.*t29.*t30.*t31.*t38.*t40.*8.0;
t473 = t6.*t7.*t10.*t12.*t14.*t19.*t29.*t30.*t31.*t38.*t40.*1.6e+1;
t474 = Gamma_w_yy.*t9.*t10.*t11.*t13.*t19.*t21.*t29.*t30.*t31.*t36.*t38.*1.6e+1;
t476 = Gamma_w_yy.*t5.*t8.*t10.*t11.*t13.*t19.*t29.*t30.*t31.*t38.*t40.*1.6e+1;
t478 = Gamma_w_yy.*t6.*t7.*t10.*t11.*t13.*t19.*t29.*t30.*t31.*t38.*t40.*3.2e+1;
t482 = Gamma_w_yy.*t7.*t10.*t11.*t13.*t19.*t22.*t29.*t30.*t31.*t36.*t38.*6.4e+1;
t45 = Gamma_b_zz.*Gamma_w_yy.*m_w.*t10.*t13.*t25.*t32.*t34.*t41.*4.0;
t47 = Gamma_w_yy.*Gamma_w_zz.*m_w.*t10.*t13.*t25.*t32.*t34.*t41.*8.0;
t48 = m_w.*t2.*t7.*t10.*t19.*t32.*t40.*t41.*4.0;
t50 = Gamma_b_zz.*t10.*t11.*t14.*t25.*t32.*t34.*t41.*4.0;
t52 = Gamma_b_yy.*Gamma_b_zz.*Gamma_w_yy.*t13.*t24.*t25.*t30.*t34.*t41.*4.0;
t55 = Gamma_b_yy.*Gamma_b_zz.*m_w.*t14.*t24.*t25.*t30.*t34.*t41.*4.0;
t59 = Gamma_w_zz.*t10.*t11.*t14.*t25.*t32.*t34.*t41.*8.0;
t61 = Gamma_b_yy.*Gamma_w_yy.*Gamma_w_zz.*t13.*t24.*t25.*t30.*t34.*t41.*8.0;
t62 = Gamma_b_yy.*t2.*t7.*t19.*t24.*t30.*t40.*t41.*4.0;
t65 = Gamma_b_zz.*Gamma_w_yy.*m_w.*t5.*t10.*t13.*t17.*t32.*t34.*t41.*8.0;
t69 = Gamma_w_yy.*Gamma_w_zz.*m_w.*t5.*t10.*t13.*t17.*t32.*t34.*t41.*1.6e+1;
t72 = m_w.*t2.*t5.*t8.*t10.*t19.*t32.*t36.*t41.*4.0;
t76 = Gamma_b_yy.*Gamma_w_zz.*m_w.*t14.*t24.*t25.*t30.*t34.*t41.*8.0;
t79 = Gamma_b_yy.*Gamma_b_zz.*m_w.*t5.*t14.*t17.*t24.*t30.*t34.*t41.*8.0;
t85 = Gamma_b_yy.*Gamma_w_zz.*m_w.*t5.*t14.*t17.*t24.*t30.*t34.*t41.*1.6e+1;
t89 = -t57;
t99 = Gamma_b_yy.*Gamma_w_yy.*m_w.*t7.*t13.*t19.*t24.*t32.*t34.*t41;
t100 = -t63;
t102 = -t73;
t103 = m_w.*t2.*t6.*t7.*t10.*t19.*t32.*t36.*t41.*8.0;
t106 = Gamma_b_zz.*t5.*t10.*t11.*t14.*t17.*t32.*t34.*t41.*8.0;
t110 = Gamma_w_zz.*t5.*t10.*t11.*t14.*t17.*t32.*t34.*t41.*1.6e+1;
t115 = Gamma_b_yy.*Gamma_b_zz.*Gamma_w_yy.*t5.*t13.*t17.*t24.*t30.*t34.*t41.*8.0;
t119 = Gamma_b_yy.*Gamma_w_yy.*Gamma_w_zz.*t5.*t13.*t17.*t24.*t30.*t34.*t41.*1.6e+1;
t122 = Gamma_b_yy.*t2.*t5.*t8.*t19.*t24.*t30.*t36.*t41.*4.0;
t128 = t7.*t10.*t12.*t14.*t19.*t32.*t40.*t41.*4.0;
t137 = -t91;
t142 = -t93;
t154 = t5.*t8.*t10.*t12.*t14.*t19.*t32.*t36.*t41.*4.0;
t157 = Gamma_b_yy.*Gamma_b_zz.*Gamma_w_yy.*t13.*t15.*t16.*t25.*t30.*t34.*t41.*8.0;
t159 = Gamma_b_yy.*Gamma_w_yy.*Gamma_w_zz.*t13.*t15.*t16.*t25.*t30.*t34.*t41.*1.6e+1;
t160 = -t95;
t175 = Gamma_b_yy.*Gamma_b_zz.*m_w.*t14.*t15.*t16.*t25.*t30.*t34.*t41.*8.0;
t178 = Gamma_b_yy.*Gamma_w_zz.*m_w.*t14.*t15.*t16.*t25.*t30.*t34.*t41.*1.6e+1;
t179 = -t97;
t185 = Gamma_b_yy.*t7.*t11.*t14.*t19.*t24.*t32.*t34.*t41;
t188 = -t113;
t190 = -t123;
t191 = Gamma_b_yy.*t2.*t6.*t7.*t19.*t24.*t30.*t36.*t41.*8.0;
t193 = -t130;
t194 = -t132;
t195 = -t139;
t196 = -t141;
t197 = -t144;
t198 = -t149;
t200 = -t151;
t201 = -t153;
t202 = Gamma_w_yy.*t7.*t10.*t11.*t13.*t19.*t32.*t40.*t41.*8.0;
t203 = -t155;
t204 = t6.*t7.*t10.*t12.*t14.*t19.*t32.*t36.*t41.*8.0;
t206 = -t162;
t207 = Gamma_b_yy.*t2.*t7.*t15.*t16.*t19.*t30.*t40.*t41.*8.0;
t208 = -t170;
t209 = -t172;
t210 = -t181;
t211 = Gamma_b_yy.*Gamma_w_yy.*m_w.*t7.*t13.*t19.*t24.*t30.*t40.*t41.*8.0;
t213 = Gamma_b_yy.*Gamma_b_zz.*Gamma_w_yy.*t5.*t13.*t15.*t16.*t17.*t30.*t34.*t41.*1.6e+1;
t217 = Gamma_b_yy.*Gamma_w_yy.*Gamma_w_zz.*t5.*t13.*t15.*t16.*t17.*t30.*t34.*t41.*3.2e+1;
t220 = Gamma_b_yy.*t7.*t11.*t14.*t19.*t24.*t30.*t40.*t41.*4.0;
t223 = Gamma_b_yy.*Gamma_b_zz.*m_w.*t5.*t14.*t15.*t16.*t17.*t30.*t34.*t41.*1.6e+1;
t229 = Gamma_b_yy.*Gamma_w_zz.*m_w.*t5.*t14.*t15.*t16.*t17.*t30.*t34.*t41.*3.2e+1;
t238 = Gamma_b_yy.*Gamma_w_yy.*m_w.*t7.*t13.*t19.*t24.*t34.*t39.*t41;
t256 = Gamma_b_yy.*Gamma_w_yy.*m_w.*t7.*t13.*t15.*t16.*t19.*t32.*t34.*t41.*2.0;
t258 = Gamma_b_yy.*Gamma_w_yy.*m_w.*t7.*t13.*t19.*t24.*t34.*t41.*t42;
t261 = Gamma_w_yy.*t5.*t8.*t10.*t11.*t13.*t19.*t32.*t36.*t41.*8.0;
t263 = Gamma_w_yy.*t6.*t7.*t10.*t11.*t13.*t19.*t32.*t36.*t41.*1.6e+1;
t267 = Gamma_b_yy.*t2.*t5.*t8.*t15.*t16.*t19.*t30.*t36.*t41.*8.0;
t269 = Gamma_b_yy.*t2.*t6.*t7.*t15.*t16.*t19.*t30.*t36.*t41.*1.6e+1;
t273 = -t187;
t274 = Gamma_b_yy.*Gamma_w_yy.*m_w.*t5.*t8.*t13.*t19.*t24.*t30.*t36.*t41.*8.0;
t276 = Gamma_b_yy.*Gamma_w_yy.*m_w.*t6.*t7.*t13.*t19.*t24.*t30.*t36.*t41.*1.6e+1;
t288 = Gamma_b_yy.*t7.*t11.*t14.*t19.*t24.*t34.*t39.*t41;
t291 = Gamma_b_yy.*t5.*t8.*t11.*t14.*t19.*t24.*t30.*t36.*t41.*4.0;
t300 = -t244;
t301 = -t246;
t303 = -t250;
t304 = -t252;
t305 = Gamma_b_yy.*Gamma_w_yy.*m_w.*t7.*t13.*t15.*t16.*t19.*t30.*t40.*t41.*1.6e+1;
t309 = Gamma_b_yy.*t7.*t11.*t14.*t15.*t16.*t19.*t32.*t34.*t41.*2.0;
t311 = Gamma_b_yy.*t7.*t11.*t14.*t19.*t24.*t34.*t41.*t42;
t313 = -t259;
t317 = Gamma_b_yy.*Gamma_w_yy.*m_w.*t6.*t7.*t13.*t15.*t16.*t19.*t29.*t34.*t41.*4.0;
t324 = -t262;
t325 = -t265;
t326 = -t268;
t327 = -t271;
t328 = -t275;
t329 = -t280;
t333 = -t284;
t334 = -t286;
t335 = -t242;
t336 = -t292;
t337 = Gamma_b_yy.*t6.*t7.*t11.*t14.*t19.*t24.*t30.*t36.*t41.*8.0;
t339 = -t294;
t340 = -t296;
t345 = Gamma_b_yy.*t7.*t11.*t14.*t15.*t16.*t19.*t30.*t40.*t41.*8.0;
t350 = -t315;
t351 = Gamma_b_yy.*Gamma_w_yy.*m_w.*t5.*t8.*t13.*t15.*t16.*t19.*t30.*t36.*t41.*1.6e+1;
t353 = Gamma_b_yy.*Gamma_w_yy.*m_w.*t6.*t7.*t13.*t15.*t16.*t19.*t30.*t36.*t41.*3.2e+1;
t359 = Gamma_b_yy.*t6.*t7.*t11.*t14.*t15.*t16.*t19.*t29.*t34.*t41.*4.0;
t369 = Gamma_b_yy.*Gamma_w_yy.*m_w.*t7.*t13.*t15.*t16.*t19.*t23.*t29.*t34.*t41.*4.0;
t372 = -t348;
t374 = -t352;
t379 = -t357;
t380 = Gamma_b_yy.*t5.*t8.*t11.*t14.*t15.*t16.*t19.*t30.*t36.*t41.*8.0;
t382 = Gamma_b_yy.*t6.*t7.*t11.*t14.*t15.*t16.*t19.*t30.*t36.*t41.*1.6e+1;
t385 = -t367;
t389 = Gamma_b_yy.*t7.*t11.*t14.*t15.*t16.*t19.*t23.*t29.*t34.*t41.*4.0;
t390 = -t371;
t395 = -t377;
t396 = -t381;
t397 = -t387;
t398 = -t394;
t402 = Gamma_b_zz.*Gamma_w_yy.*m_w.*t10.*t13.*t25.*t29.*t30.*t31.*t34.*t41.*8.0;
t404 = Gamma_w_yy.*Gamma_w_zz.*m_w.*t10.*t13.*t25.*t29.*t30.*t31.*t34.*t41.*1.6e+1;
t405 = m_w.*t2.*t7.*t10.*t19.*t29.*t30.*t31.*t40.*t41.*8.0;
t407 = Gamma_b_zz.*t10.*t11.*t14.*t25.*t29.*t30.*t31.*t34.*t41.*8.0;
t409 = Gamma_w_zz.*t10.*t11.*t14.*t25.*t29.*t30.*t31.*t34.*t41.*1.6e+1;
t411 = Gamma_b_zz.*Gamma_w_yy.*m_w.*t5.*t10.*t13.*t17.*t29.*t30.*t31.*t34.*t41.*1.6e+1;
t415 = Gamma_w_yy.*Gamma_w_zz.*m_w.*t5.*t10.*t13.*t17.*t29.*t30.*t31.*t34.*t41.*3.2e+1;
t420 = m_w.*t2.*t5.*t8.*t10.*t19.*t29.*t30.*t31.*t36.*t41.*8.0;
t422 = m_w.*t2.*t6.*t7.*t10.*t19.*t29.*t30.*t31.*t36.*t41.*1.6e+1;
t425 = Gamma_b_zz.*t5.*t10.*t11.*t14.*t17.*t29.*t30.*t31.*t34.*t41.*1.6e+1;
t429 = Gamma_w_zz.*t5.*t10.*t11.*t14.*t17.*t29.*t30.*t31.*t34.*t41.*3.2e+1;
t442 = -t418;
t443 = -t421;
t446 = t7.*t10.*t12.*t14.*t19.*t29.*t30.*t31.*t40.*t41.*8.0;
t447 = -t435;
t448 = -t437;
t451 = -t439;
t452 = -t441;
t463 = -t454;
t464 = -t456;
t465 = -t458;
t466 = -t460;
t469 = Gamma_w_yy.*t7.*t10.*t11.*t13.*t19.*t29.*t30.*t31.*t40.*t41.*1.6e+1;
t470 = t5.*t8.*t10.*t12.*t14.*t19.*t29.*t30.*t31.*t36.*t41.*8.0;
t472 = t6.*t7.*t10.*t12.*t14.*t19.*t29.*t30.*t31.*t36.*t41.*1.6e+1;
t475 = Gamma_w_yy.*t5.*t8.*t10.*t11.*t13.*t19.*t29.*t30.*t31.*t36.*t41.*1.6e+1;
t477 = Gamma_w_yy.*t6.*t7.*t10.*t11.*t13.*t19.*t29.*t30.*t31.*t36.*t41.*3.2e+1;
t479 = -t467;
t480 = -t471;
t481 = -t474;
t483 = -t476;
et1 = t44+t45+t46+t47+t48+t49+t50+t51+t52+t53+t54+t55+t56+t58+t59+t60+t61+t62+t64+t65+t66+t67+t68+t69+t70+t71+t72+t74+t75+t76+t77+t78+t79+t80+t81+t82+t83+t84+t85+t86+t87+t88+t89+t90+t92+t94+t96+t98+t99+t100+t101+t102+t103+t104+t105+t106+t107+t108+t109+t110+t111+t112+t114+t115+t116+t117+t118+t119+t120+t121+t122+t124+t125+t126+t127+t128+t129+t131+t133+t134+t135+t136+t137+t138+t140+t142+t143+t145+t146+t147+t148+t150+t152+t154+t156+t157+t158+t159+t160+t161+t163+t164+t165+t166+t167+t168+t169+t171+t173+t174+t175+t176+t177+t178+t179+t180+t182+t183+t184+t185+t186+t188+t189+t190+t191+t192+t193+t194+t195+t196+t197+t198+t199+t200+t201+t202+t203+t204+t205+t206+t207+t208+t209+t210+t211+t212+t213+t214+t215+t216+t217+t218+t219+t220+t221+t222+t223+t224+t225+t226+t227+t228+t229+t230+t231+t232+t233+t234+t235+t236+t237+t238+t239+t240+t241+t243+t245+t247+t249+t251+t253+t254+t255+t256+t257+t258+t260+t261+t263+t264+t266+t267+t269+t270+t272+t273+t274+t276+t277+t278;
et2 = t279+t281+t282+t283+t285+t287+t288+t289+t290+t291+t293+t295+t297+t298+t299+t300+t301+t302+t303+t304+t305+t306+t308+t309+t310+t311+t312+t313+t314+t316+t317+t318+t319+t320+t322+t323+t324+t325+t326+t327+t328+t329+t330+t331+t332+t333+t334+t335+t336+t337+t338+t339+t340+t341+t342+t343+t344+t345+t346+t347+t349+t350+t351+t353+t354+t355+t356+t358+t359+t360+t361+t362+t364+t365+t366+t368+t369+t370+t372+t373+t374+t375+t376+t378+t379+t380+t382+t383+t384+t385+t386+t388+t389+t390+t391+t392+t393+t395+t396+t397+t398+t399+t400+t401+t402+t403+t404+t405+t406+t407+t408+t409+t410+t411+t412+t413+t414+t415+t416+t417+t419+t420+t422+t423+t424+t425+t426+t427+t428+t429+t430+t431+t432+t433+t434+t436+t438+t440+t442+t443+t444+t445+t446+t447+t448+t449+t450+t451+t452+t453+t455+t457+t459+t461+t462+t463+t464+t465+t466+t468+t469+t470+t472+t473+t475+t477+t478+t479+t480+t481+t482+t483;
t484 = et1+et2;
t485 = 1.0./t484;
et3 = t2.*t7.*t19.*t30.*t40.*t41.*4.0+Gamma_b_zz.*Gamma_w_yy.*t13.*t25.*t30.*t34.*t41.*4.0+Gamma_b_zz.*Gamma_w_yy.*t13.*t25.*t30.*t37.*t40.*4.0+Gamma_w_yy.*Gamma_w_zz.*t13.*t25.*t30.*t34.*t41.*8.0+Gamma_w_yy.*Gamma_w_zz.*t13.*t25.*t30.*t37.*t40.*8.0+Gamma_b_zz.*m_w.*t14.*t25.*t32.*t34.*t37.*4.0+Gamma_b_zz.*m_w.*t14.*t25.*t30.*t34.*t41.*4.0+Gamma_b_zz.*m_w.*t14.*t25.*t30.*t37.*t40.*4.0+Gamma_w_zz.*m_w.*t14.*t25.*t32.*t34.*t37.*8.0+Gamma_w_zz.*m_w.*t14.*t25.*t30.*t34.*t41.*8.0+Gamma_w_zz.*m_w.*t14.*t25.*t30.*t37.*t40.*8.0+t2.*t5.*t8.*t19.*t30.*t36.*t41.*4.0+t2.*t6.*t7.*t19.*t30.*t36.*t41.*8.0-t2.*t5.*t8.*t19.*t30.*t38.*t40.*4.0+t2.*t6.*t7.*t19.*t30.*t38.*t40.*8.0+t2.*t7.*t19.*t22.*t30.*t36.*t38.*1.6e+1-t2.*t9.*t19.*t21.*t30.*t36.*t38.*4.0+t7.*t11.*t14.*t19.*t32.*t34.*t41+t7.*t11.*t14.*t19.*t32.*t37.*t40+t7.*t11.*t14.*t19.*t30.*t40.*t41.*4.0+t7.*t11.*t14.*t19.*t34.*t39.*t41;
et4 = t7.*t11.*t14.*t19.*t37.*t39.*t40+t7.*t11.*t14.*t19.*t34.*t41.*t42+t7.*t11.*t14.*t19.*t37.*t40.*t42+Gamma_b_zz.*Gamma_w_yy.*t5.*t13.*t17.*t30.*t34.*t41.*8.0+Gamma_b_zz.*Gamma_w_yy.*t5.*t13.*t17.*t30.*t37.*t40.*8.0+Gamma_b_zz.*Gamma_w_yy.*t6.*t13.*t25.*t30.*t34.*t38.*8.0+Gamma_b_zz.*Gamma_w_yy.*t6.*t13.*t25.*t30.*t36.*t37.*8.0+Gamma_w_yy.*Gamma_w_zz.*t5.*t13.*t17.*t30.*t34.*t41.*1.6e+1+Gamma_w_yy.*Gamma_w_zz.*t5.*t13.*t17.*t30.*t37.*t40.*1.6e+1+Gamma_w_yy.*Gamma_w_zz.*t6.*t13.*t25.*t30.*t34.*t38.*1.6e+1+Gamma_w_yy.*Gamma_w_zz.*t6.*t13.*t25.*t30.*t36.*t37.*1.6e+1+Gamma_b_zz.*m_w.*t5.*t14.*t17.*t32.*t34.*t37.*8.0+Gamma_b_zz.*m_w.*t5.*t14.*t17.*t30.*t34.*t41.*8.0+Gamma_b_zz.*m_w.*t5.*t14.*t17.*t30.*t37.*t40.*8.0+Gamma_b_zz.*m_w.*t6.*t14.*t25.*t29.*t34.*t37.*8.0+Gamma_b_zz.*m_w.*t6.*t14.*t25.*t30.*t34.*t38.*8.0+Gamma_b_zz.*m_w.*t6.*t14.*t25.*t30.*t36.*t37.*8.0+Gamma_w_zz.*m_w.*t5.*t14.*t17.*t32.*t34.*t37.*1.6e+1+Gamma_b_zz.*m_w.*t14.*t23.*t25.*t29.*t34.*t37.*8.0;
et5 = Gamma_w_zz.*m_w.*t5.*t14.*t17.*t30.*t34.*t41.*1.6e+1+Gamma_w_zz.*m_w.*t5.*t14.*t17.*t30.*t37.*t40.*1.6e+1+Gamma_w_yy.*m_w.*t7.*t13.*t19.*t32.*t34.*t41+Gamma_w_zz.*m_w.*t6.*t14.*t25.*t29.*t34.*t37.*1.6e+1+Gamma_w_yy.*m_w.*t7.*t13.*t19.*t32.*t37.*t40+Gamma_w_zz.*m_w.*t6.*t14.*t25.*t30.*t34.*t38.*1.6e+1+Gamma_w_yy.*m_w.*t7.*t13.*t19.*t30.*t40.*t41.*8.0+Gamma_w_zz.*m_w.*t6.*t14.*t25.*t30.*t36.*t37.*1.6e+1+Gamma_w_yy.*m_w.*t7.*t13.*t19.*t34.*t39.*t41+Gamma_w_yy.*m_w.*t7.*t13.*t19.*t37.*t39.*t40+Gamma_w_yy.*m_w.*t7.*t13.*t19.*t34.*t41.*t42+Gamma_w_yy.*m_w.*t7.*t13.*t19.*t37.*t40.*t42+Gamma_w_zz.*m_w.*t14.*t23.*t25.*t29.*t34.*t37.*1.6e+1-t5.*t8.*t11.*t14.*t19.*t32.*t34.*t38+t6.*t7.*t11.*t14.*t19.*t32.*t34.*t38.*2.0+t5.*t8.*t11.*t14.*t19.*t32.*t36.*t37+t6.*t7.*t11.*t14.*t19.*t32.*t36.*t37.*2.0+t5.*t8.*t11.*t14.*t19.*t30.*t36.*t41.*4.0+t6.*t7.*t11.*t14.*t19.*t30.*t36.*t41.*8.0;
et6 = t5.*t8.*t11.*t14.*t19.*t30.*t38.*t40.*-4.0+t6.*t7.*t11.*t14.*t19.*t30.*t38.*t40.*8.0+t5.*t8.*t11.*t14.*t19.*t36.*t37.*t39+t5.*t8.*t11.*t14.*t19.*t36.*t37.*t42+t7.*t11.*t14.*t19.*t22.*t29.*t34.*t38.*4.0+t7.*t11.*t14.*t19.*t22.*t29.*t36.*t37.*4.0+t7.*t11.*t14.*t19.*t22.*t30.*t36.*t38.*1.6e+1-t9.*t11.*t14.*t19.*t21.*t30.*t36.*t38.*4.0-Gamma_b_zz.*Gamma_w_yy.*d.*t5.*t13.*t25.*t30.*t34.*t38.*4.0+Gamma_b_zz.*Gamma_w_yy.*d.*t5.*t13.*t25.*t30.*t36.*t37.*4.0-Gamma_b_zz.*Gamma_w_yy.*d.*t13.*t17.*t21.*t30.*t34.*t38.*8.0+Gamma_b_zz.*Gamma_w_yy.*d.*t13.*t17.*t21.*t30.*t36.*t37.*8.0-Gamma_w_yy.*Gamma_w_zz.*d.*t5.*t13.*t25.*t30.*t34.*t38.*8.0+Gamma_w_yy.*Gamma_w_zz.*d.*t5.*t13.*t25.*t30.*t36.*t37.*8.0-Gamma_w_yy.*Gamma_w_zz.*d.*t13.*t17.*t21.*t30.*t34.*t38.*1.6e+1+Gamma_w_yy.*Gamma_w_zz.*d.*t13.*t17.*t21.*t30.*t36.*t37.*1.6e+1+Gamma_b_zz.*Gamma_w_yy.*t5.*t6.*t13.*t17.*t30.*t34.*t38.*1.6e+1;
et7 = Gamma_b_zz.*Gamma_w_yy.*t5.*t6.*t13.*t17.*t30.*t36.*t37.*1.6e+1+Gamma_w_yy.*Gamma_w_zz.*t5.*t6.*t13.*t17.*t30.*t34.*t38.*3.2e+1+Gamma_w_yy.*Gamma_w_zz.*t5.*t6.*t13.*t17.*t30.*t36.*t37.*3.2e+1-Gamma_b_zz.*d.*m_w.*t5.*t14.*t25.*t30.*t34.*t38.*4.0+Gamma_b_zz.*d.*m_w.*t5.*t14.*t25.*t30.*t36.*t37.*4.0-Gamma_b_zz.*d.*m_w.*t14.*t17.*t21.*t30.*t34.*t38.*8.0+Gamma_b_zz.*d.*m_w.*t14.*t17.*t21.*t30.*t36.*t37.*8.0-Gamma_w_zz.*d.*m_w.*t5.*t14.*t25.*t30.*t34.*t38.*8.0+Gamma_w_zz.*d.*m_w.*t5.*t14.*t25.*t30.*t36.*t37.*8.0-Gamma_w_zz.*d.*m_w.*t14.*t17.*t21.*t30.*t34.*t38.*1.6e+1+Gamma_w_zz.*d.*m_w.*t14.*t17.*t21.*t30.*t36.*t37.*1.6e+1+Gamma_b_zz.*m_w.*t5.*t6.*t14.*t17.*t29.*t34.*t37.*1.6e+1+Gamma_b_zz.*m_w.*t5.*t6.*t14.*t17.*t30.*t34.*t38.*1.6e+1+Gamma_b_zz.*m_w.*t5.*t6.*t14.*t17.*t30.*t36.*t37.*1.6e+1+Gamma_b_zz.*m_w.*t5.*t14.*t17.*t23.*t29.*t34.*t37.*1.6e+1+Gamma_w_zz.*m_w.*t5.*t6.*t14.*t17.*t29.*t34.*t37.*3.2e+1;
et8 = Gamma_w_zz.*m_w.*t5.*t6.*t14.*t17.*t30.*t34.*t38.*3.2e+1+Gamma_w_zz.*m_w.*t5.*t6.*t14.*t17.*t30.*t36.*t37.*3.2e+1-Gamma_w_yy.*m_w.*t5.*t8.*t13.*t19.*t32.*t34.*t38+Gamma_w_yy.*m_w.*t6.*t7.*t13.*t19.*t32.*t34.*t38.*2.0+Gamma_w_yy.*m_w.*t5.*t8.*t13.*t19.*t32.*t36.*t37+Gamma_w_yy.*m_w.*t6.*t7.*t13.*t19.*t32.*t36.*t37.*2.0+Gamma_w_yy.*m_w.*t5.*t8.*t13.*t19.*t30.*t36.*t41.*8.0+Gamma_w_yy.*m_w.*t6.*t7.*t13.*t19.*t30.*t36.*t41.*1.6e+1-Gamma_w_yy.*m_w.*t5.*t8.*t13.*t19.*t30.*t38.*t40.*8.0+Gamma_w_yy.*m_w.*t6.*t7.*t13.*t19.*t30.*t38.*t40.*1.6e+1+Gamma_w_yy.*m_w.*t5.*t8.*t13.*t19.*t36.*t37.*t39+Gamma_w_yy.*m_w.*t5.*t8.*t13.*t19.*t36.*t37.*t42+Gamma_w_zz.*m_w.*t5.*t14.*t17.*t23.*t29.*t34.*t37.*3.2e+1+Gamma_w_yy.*m_w.*t7.*t13.*t19.*t22.*t29.*t34.*t38.*4.0+Gamma_w_yy.*m_w.*t7.*t13.*t19.*t22.*t29.*t36.*t37.*4.0+Gamma_w_yy.*m_w.*t7.*t13.*t19.*t22.*t30.*t36.*t38.*3.2e+1-Gamma_w_yy.*m_w.*t9.*t13.*t19.*t21.*t30.*t36.*t38.*8.0;
et9 = t5.*t6.*t8.*t11.*t14.*t19.*t29.*t34.*t38.*-2.0-t5.*t8.*t11.*t14.*t19.*t23.*t29.*t34.*t38.*2.0+t6.*t7.*t11.*t14.*t19.*t23.*t29.*t34.*t38.*4.0+t6.*t7.*t11.*t14.*t19.*t23.*t29.*t36.*t37.*4.0-Gamma_w_yy.*m_w.*t5.*t6.*t8.*t13.*t19.*t29.*t34.*t38.*2.0-Gamma_w_yy.*m_w.*t5.*t8.*t13.*t19.*t23.*t29.*t34.*t38.*2.0+Gamma_w_yy.*m_w.*t6.*t7.*t13.*t19.*t23.*t29.*t34.*t38.*4.0+Gamma_w_yy.*m_w.*t6.*t7.*t13.*t19.*t23.*t29.*t36.*t37.*4.0;
mt1 = [t6,-g.*m_w.*t10.*t13.*t20.*t43.*t485.*(Gamma_b_zz.*t13.*t25.*t34.*t37.*4.0+Gamma_w_yy.*t7.*t19.*t34.*t41+Gamma_w_yy.*t7.*t19.*t37.*t40+Gamma_w_zz.*t13.*t25.*t34.*t37.*8.0+m_w.*t7.*t13.*t19.*t34.*t41+m_w.*t7.*t13.*t19.*t37.*t40+Gamma_b_zz.*t5.*t13.*t17.*t34.*t37.*8.0-Gamma_w_yy.*t5.*t8.*t19.*t34.*t38+Gamma_w_yy.*t6.*t7.*t19.*t34.*t38.*2.0+Gamma_w_yy.*t5.*t8.*t19.*t36.*t37+Gamma_w_yy.*t6.*t7.*t19.*t36.*t37.*2.0+Gamma_w_zz.*t5.*t13.*t17.*t34.*t37.*1.6e+1-m_w.*t5.*t8.*t13.*t19.*t34.*t38+m_w.*t6.*t7.*t13.*t19.*t34.*t38.*2.0+m_w.*t5.*t8.*t13.*t19.*t36.*t37+m_w.*t6.*t7.*t13.*t19.*t36.*t37.*2.0),t4,g.*l.*t20.*t485.*(et3+et4+et5+et6+et7+et8+et9),t5];
mt2 = [g.*m_w.*t10.*t13.*t20.*t43.*t485.*(-Gamma_w_yy.*d.*t19.*t34.*t41+Gamma_w_yy.*d.*t19.*t37.*t40-d.*m_w.*t13.*t19.*t34.*t41+d.*m_w.*t13.*t19.*t37.*t40-Gamma_w_yy.*d.*t6.*t19.*t34.*t38.*2.0+Gamma_w_yy.*d.*t6.*t19.*t36.*t37.*2.0+Gamma_w_yy.*t5.*t7.*t19.*t34.*t38+Gamma_w_yy.*t5.*t7.*t19.*t36.*t37-d.*m_w.*t6.*t13.*t19.*t34.*t38.*2.0+d.*m_w.*t6.*t13.*t19.*t36.*t37.*2.0+m_w.*t5.*t7.*t13.*t19.*t34.*t38+m_w.*t5.*t7.*t13.*t19.*t36.*t37).*2.0];
dYdt = reshape([mt1,mt2],6,1);
